simulink model "three_phase_inverter"  (R2021a)
settings: Solver=ode5  StartTime=0.0  StopTime=10.0  FixedStep=1e-7  RelTol=1e-3
libraries: spsIGBTDiodeLib x6, spsSeriesRLCBranchLib x3, simulink x2, spsDCVoltageSourceLib x1, spsVoltageMeasurementLib x1, spspowerguiLib x1
settings Model: Creator=amrit  LastModifiedBy=mansi
settings SolverCC: AlgebraicLoopSolver=TrustRegion
settings DebuggingCC: SFMachineParentedDataDiag=warning

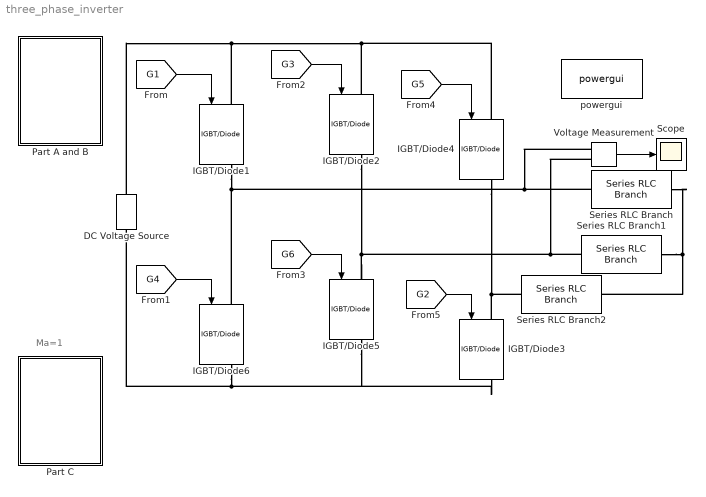
== system three_phase_inverter ==
  note: Ma=1
  DC Voltage Source : spsDCVoltageSourceLib/DC Voltage Source  Amplitude=800  Measurements=None
  IGBT/Diode{1..6} (6 alike) : spsIGBTDiodeLib/IGBT//Diode  Ron=20e-3  Rs=1e5  Cs=inf  Measurements=on
  Part A and B : Subsystem
  Part C : Subsystem
  Scope : Scope
  Series RLC Branch : spsSeriesRLCBranchLib/Series RLC Branch  LConnTagsString=__new0  RConnTagsString=__new0  BranchType=RL  Resistance=40  Inductance=20e-3  SetiL0=off  InitialCurrent=0  Capacitance=1e-6  Setx0=off  InitialVoltage=0  Measurements=None
  Series RLC Branch1 : spsSeriesRLCBranchLib/Series RLC Branch  LConnTagsString=__new0  RConnTagsString=__new0  BranchType=RL  Resistance=40  Inductance=20e-3  SetiL0=off  InitialCurrent=0  Capacitance=1e-6  Setx0=off  InitialVoltage=0  Measurements=None
  Series RLC Branch2 : spsSeriesRLCBranchLib/Series RLC Branch  LConnTagsString=__new0  RConnTagsString=__new0  BranchType=RL  Resistance=40  Inductance=20e-3  SetiL0=off  InitialCurrent=0  Capacitance=1e-6  Setx0=off  InitialVoltage=0  Measurements=None
  Voltage Measurement : spsVoltageMeasurementLib/Voltage Measurement  PhasorSimulation=off  OutputType=Complex  PSBequivalent=0
  powergui : spspowerguiLib/powergui  Priority=1  SimulationMode=Discrete  SampleTime=1e-7  frequency=60  Iterations=50  frequencyindice=60  Pbase=100e6  ErrMax=1e-4  UnitsV=kV  UnitsW=MW  buscounter=0  FunctionMessages=off  echomessages=off  EnableUseOfTLC=off  CurrentSourceSwitches=off  DisableSnubberDevices=off  DisableRonSwitches=off  DisableVfSwitches=off  DisplayEquations=off  AutomaticDiscreteSolvers=off  SolverType=Tustin/Backward Euler (TBE)  Interpol=off  ExternalGateDelay=off  methode=off  Ts=100  x0status=blocks  SPID=on  SwTol=0  HookPort=off  NonlinearTolerance=1e-4  nMaxIteration=100  ContinueOnMaxIteration=off  RestoreLinks=warning  ResistiveCurrentMeasurement=off  Frange=[0:2:500]  Ylog=off  Xlog=on  ShowGrid=off  save=off  variable=ZData  structure=0  ZoomFFT=off  StartTime=0.0  cycles=1  DisplayStyle=1  fundamental=60  FreqAxis=off  MaxFrequency=1000  frequencyindicesteady=1  RmsSteady=1  display=off
  wires:
  [G1] -> IGBT/Diode1/1
  [G4] -> IGBT/Diode6/1
  [G3] -> IGBT/Diode2/1
  [G6] -> IGBT/Diode5/1
  [G5] -> IGBT/Diode4/1
  [G2] -> IGBT/Diode3/1
  Voltage Measurement/1 -> Scope/1
  connections:
  DC Voltage Source/RConn1 -- IGBT/Diode1/LConn1 -- IGBT/Diode4/LConn1 -- IGBT/Diode2/LConn1
  Series RLC Branch/LConn1 -- Voltage Measurement/LConn1 -- IGBT/Diode6/LConn1 -- IGBT/Diode1/RConn1
  Series RLC Branch1/LConn1 -- Voltage Measurement/LConn2 -- IGBT/Diode2/RConn1 -- IGBT/Diode5/LConn1
  Series RLC Branch2/LConn1 -- IGBT/Diode4/RConn1 -- IGBT/Diode3/LConn1
  IGBT/Diode6/RConn1 -- IGBT/Diode5/RConn1 -- IGBT/Diode3/RConn1 -- DC Voltage Source/LConn1
  Series RLC Branch/RConn1 -- Series RLC Branch1/RConn1 -- Series RLC Branch2/RConn1

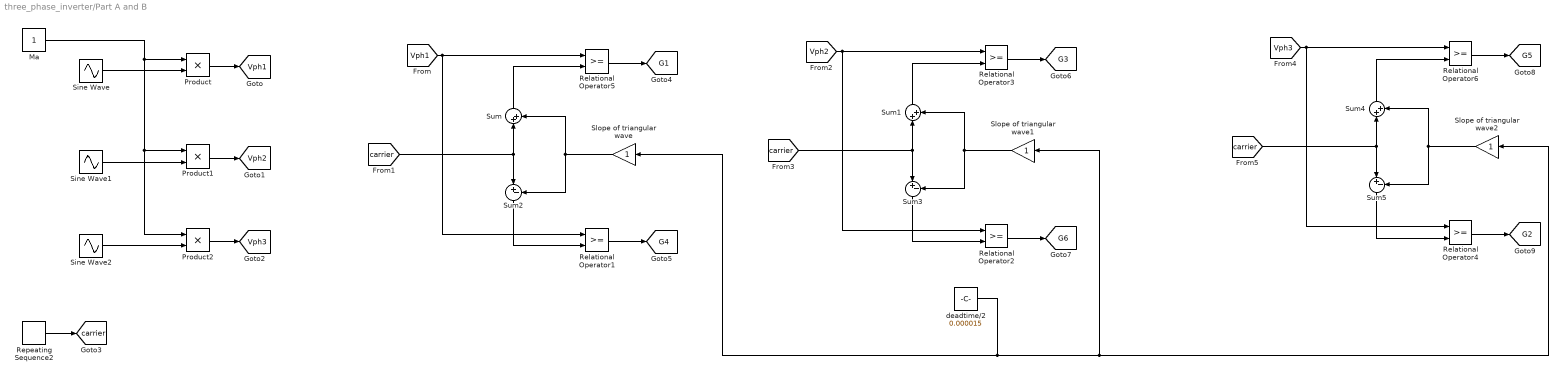
== system three_phase_inverter/Part A and B ==
  Ma : Constant
  Product : Product
  Product1 : Product
  Product2 : Product
  Relational Operator{1..6} (6 alike) : RelationalOperator  OutDataTypeStr=boolean  RndMeth=Nearest
  Repeating Sequence2 : simulink/Sources/Repeating Sequence  rep_seq_t=[0 0.0000125 0.000025 0.0000375 0.00005]  rep_seq_y=[0 1 0 -1 0]
  Sine Wave : Sin  Frequency=2*pi*60  SampleTime=0
  Sine Wave1 : Sin  Frequency=2*pi*60  Phase=-(2*pi/3)  SampleTime=0
  Sine Wave2 : Sin  Frequency=2*pi*60  Phase=2*pi/3  SampleTime=0
  Slope of triangular wave : Gain
  Slope of triangular wave1 : Gain
  Slope of triangular wave2 : Gain
  Sum : Sum  Inputs=|++
  Sum1 : Sum  Inputs=|++
  Sum2 : Sum  Inputs=|+-
  Sum3 : Sum  Inputs=|+-
  Sum4 : Sum  Inputs=|++
  Sum5 : Sum  Inputs=|+-
  deadtime/2 : Constant  Value=0.000015
  tag scope: G1=global, G2=global, G3=global, G4=global, G5=global, G6=global, Vph1=global, Vph2=global, Vph3=global, carrier=global
  wires:
  Slope of triangular wave2/1 -> Sum5/2, Sum4/2
  deadtime/2/1 -> Slope of triangular wave1/1, Slope of triangular wave2/1, Slope of triangular wave/1
  Sum4/1 -> Relational Operator6/2
  Ma/1 -> Product2/1, Product1/1, Product/1
  [carrier] -> Sum2/1, Sum/1
  Product2/1 -> [Vph3]
  Product1/1 -> [Vph2]
  [Vph1] -> Relational Operator1/1, Relational Operator5/1
  [Vph3] -> Relational Operator4/1, Relational Operator6/1
  Slope of triangular wave1/1 -> Sum3/2, Sum1/2
  [carrier] -> Sum5/1, Sum4/1
  Sum1/1 -> Relational Operator3/2
  Relational Operator1/1 -> [G4]
  [carrier] -> Sum3/1, Sum1/1
  Sine Wave/1 -> Product/2
  Sum5/1 -> Relational Operator4/2
  Relational Operator4/1 -> [G2]
  Slope of triangular wave/1 -> Sum2/2, Sum/2
  Relational Operator6/1 -> [G5]
  Sine Wave2/1 -> Product2/2
  Relational Operator3/1 -> [G3]
  Sum2/1 -> Relational Operator1/2
  Relational Operator2/1 -> [G6]
  Sine Wave1/1 -> Product1/2
  Sum/1 -> Relational Operator5/2
  Product/1 -> [Vph1]
  Repeating Sequence2/1 -> [carrier]
  Sum3/1 -> Relational Operator2/2
  [Vph2] -> Relational Operator2/1, Relational Operator3/1
  Relational Operator5/1 -> [G1]

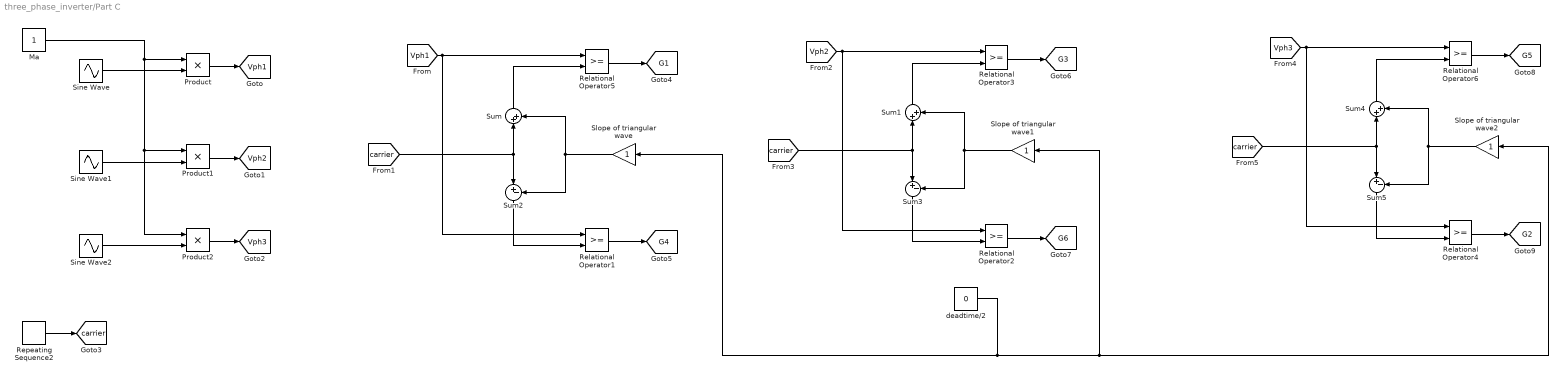
== system three_phase_inverter/Part C ==
  Ma : Constant
  Product : Product
  Product1 : Product
  Product2 : Product
  Relational Operator{1..6} (6 alike) : RelationalOperator  OutDataTypeStr=boolean  RndMeth=Nearest
  Repeating Sequence2 : simulink/Sources/Repeating Sequence  rep_seq_t=[0 0.0000125 0.000025 0.0000375 0.00005]  rep_seq_y=[0 1 0 -1 0]
  Sine Wave : Sin  Frequency=2*pi*60  SampleTime=0
  Sine Wave1 : Sin  Frequency=2*pi*60  Phase=-(2*pi/3)  SampleTime=0
  Sine Wave2 : Sin  Frequency=2*pi*60  Phase=2*pi/3  SampleTime=0
  Slope of triangular wave : Gain
  Slope of triangular wave1 : Gain
  Slope of triangular wave2 : Gain
  Sum : Sum  Inputs=|++
  Sum1 : Sum  Inputs=|++
  Sum2 : Sum  Inputs=|+-
  Sum3 : Sum  Inputs=|+-
  Sum4 : Sum  Inputs=|++
  Sum5 : Sum  Inputs=|+-
  deadtime/2 : Constant  Value=0
  tag scope: G1=global, G2=global, G3=global, G4=global, G5=global, G6=global, Vph1=global, Vph2=global, Vph3=global, carrier=global
  wires:
  Slope of triangular wave2/1 -> Sum5/2, Sum4/2
  deadtime/2/1 -> Slope of triangular wave1/1, Slope of triangular wave2/1, Slope of triangular wave/1
  Sum4/1 -> Relational Operator6/2
  Ma/1 -> Product2/1, Product1/1, Product/1
  [carrier] -> Sum2/1, Sum/1
  Product2/1 -> [Vph3]
  Product1/1 -> [Vph2]
  [Vph1] -> Relational Operator1/1, Relational Operator5/1
  [Vph3] -> Relational Operator4/1, Relational Operator6/1
  Slope of triangular wave1/1 -> Sum3/2, Sum1/2
  [carrier] -> Sum5/1, Sum4/1
  Sum1/1 -> Relational Operator3/2
  Relational Operator1/1 -> [G4]
  [carrier] -> Sum3/1, Sum1/1
  Sine Wave/1 -> Product/2
  Sum5/1 -> Relational Operator4/2
  Relational Operator4/1 -> [G2]
  Slope of triangular wave/1 -> Sum2/2, Sum/2
  Relational Operator6/1 -> [G5]
  Sine Wave2/1 -> Product2/2
  Relational Operator3/1 -> [G3]
  Sum2/1 -> Relational Operator1/2
  Relational Operator2/1 -> [G6]
  Sine Wave1/1 -> Product1/2
  Sum/1 -> Relational Operator5/2
  Product/1 -> [Vph1]
  Repeating Sequence2/1 -> [carrier]
  Sum3/1 -> Relational Operator2/2
  [Vph2] -> Relational Operator2/1, Relational Operator3/1
  Relational Operator5/1 -> [G1]
